simulink model "Radar_V1"  (R2018a)
settings: configuration reference "Config_Ctrl" (kept outside this file)
PreLoadFcn:
  | Radar_V1_BusInfo;
libraries: simulink x2
settings Model: Creator=IAEC nishito  LastModifiedBy=E00026
settings ConfigSetRef: SourceLocation=Base Workspace

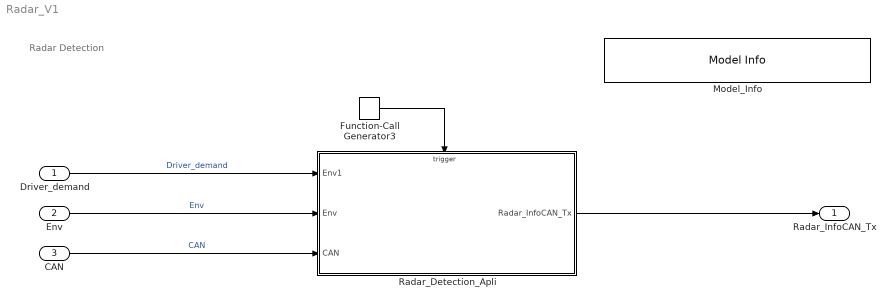
== system Radar_V1 ==
  note: Radar Detection
  Driver_demand : Inport  OutDataTypeStr=Bus: Driver_demand_Bus
      settings: AttributesFormatString=<%<OutDataTypeStr>>
  Env : Inport  Port=2  OutDataTypeStr=Bus: Environment_Bus
      settings: AttributesFormatString=<%<OutDataTypeStr>>
  CAN : Inport  Port=3  OutDataTypeStr=Bus: CAN_Bus
      settings: AttributesFormatString=<%<OutDataTypeStr>>
  Function-Call Generator3 : simulink/Ports & Subsystems/Function-Call Generator  sample_time=0.1  numberOfIterations=1
      settings: AttributesFormatString=<sample_time=%<sample_time>>
  Model_Info : simulink/Model-Wide Utilities/Model Info  Frame=on  DisplayStringWithTags=|  HorizontalTextAlignment=Left  LeftAlignmentValue=0.02
      | Version  %<ModelVersion>
      | LastModifided by %<LastModifiedBy>  Date %<LastModificationDate>
      | Description  %<Description>
  Radar_Detection_Apli : Subsystem
  Radar_InfoCAN_Tx : Outport  OutDataTypeStr=Bus: Radar_InfoCAN_Tx_Bus
      settings: AttributesFormatString=<%<OutDataTypeStr>>
  wires:
  Radar_Detection_Apli/1(Radar_InfoCAN_Tx) -> Radar_InfoCAN_Tx/1
  CAN/1 -> Radar_Detection_Apli/3(CAN)  "CAN"
  Env/1 -> Radar_Detection_Apli/2(Env)  "Env"
  Function-Call Generator3/1 -> Radar_Detection_Apli/Trigger
  Driver_demand/1 -> Radar_Detection_Apli/1(Env1)  "Driver_demand"

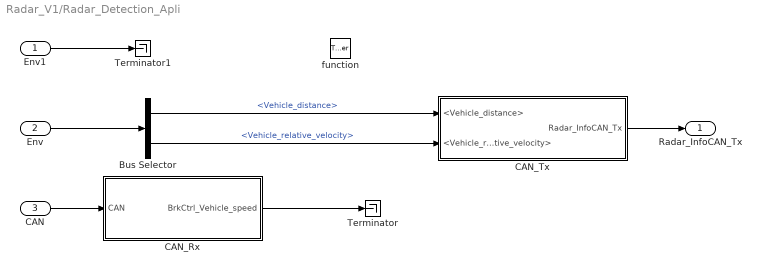
== system Radar_V1/Radar_Detection_Apli ==
  Env1 : Inport
  Env : Inport  Port=2
  CAN : Inport  Port=3
  function : TriggerPort  TriggerType=function-call  VariantControl=Variant
  Bus Selector : BusSelector  OutputSignals=Vehicle_distance,Vehicle_relative_velocity
  CAN_Rx : Subsystem
  CAN_Tx : Subsystem
  Terminator : Terminator
  Terminator1 : Terminator
  Radar_InfoCAN_Tx : Outport
  wires:
  Env/1 -> Bus Selector/1
  Bus Selector/1 -> CAN_Tx/1(<Vehicle_distance>)  "<Vehicle_distance>"
  Bus Selector/2 -> CAN_Tx/2(<Vehicle_relative_velocity>)  "<Vehicle_relative_velocity>"
  CAN_Tx/1(Radar_InfoCAN_Tx) -> Radar_InfoCAN_Tx/1
  CAN/1 -> CAN_Rx/1(CAN)
  CAN_Rx/1(BrkCtrl_Vehicle_speed) -> Terminator/1
  Env1/1 -> Terminator1/1

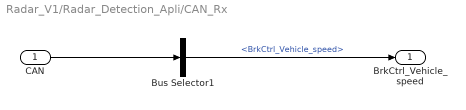
== system Radar_V1/Radar_Detection_Apli/CAN_Rx ==
  CAN : Inport
  Bus Selector1 : BusSelector  OutputSignals=VehCAN.BrakeCtrl_VehCAN_Tx.BrkCtrl_Vehicle_speed
  BrkCtrl_Vehicle_speed : Outport
  wires:
  CAN/1 -> Bus Selector1/1
  Bus Selector1/1 -> BrkCtrl_Vehicle_speed/1  "<BrkCtrl_Vehicle_speed>"

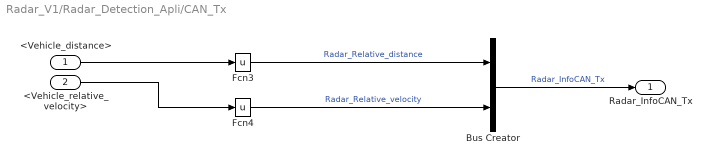
== system Radar_V1/Radar_Detection_Apli/CAN_Tx ==
  <Vehicle_distance> : Inport
  <Vehicle_relative_velocity> : Inport  Port=2
  Bus Creator : BusCreator  Inputs=2  OutDataTypeStr=Bus: Radar_InfoCAN_Tx_Bus
      settings: AttributesFormatString=<%<OutDataTypeStr>>
  Fcn3 : Fcn  Expr=u
  Fcn4 : Fcn  Expr=u
  Radar_InfoCAN_Tx : Outport
  wires:
  Fcn4/1 -> Bus Creator/2  "Radar_Relative_velocity"
  Fcn3/1 -> Bus Creator/1  "Radar_Relative_distance"
  Bus Creator/1 -> Radar_InfoCAN_Tx/1  "Radar_InfoCAN_Tx"
  <Vehicle_distance>/1 -> Fcn3/1
  <Vehicle_relative_velocity>/1 -> Fcn4/1
